simulink model "gabelstapler_Simulink"  (R2025a)
settings: Solver=VariableStepAuto  StartTime=0.0  StopTime=100  RelTol=1e-3
undefined symbols (not defined in the file): d_gtr, k_e, k_Motor, L_Motor, m_fz, m_gabel, R_Motor, r_R, theta_red
settings Model: Creator=Manuel  LastModifiedBy=baier

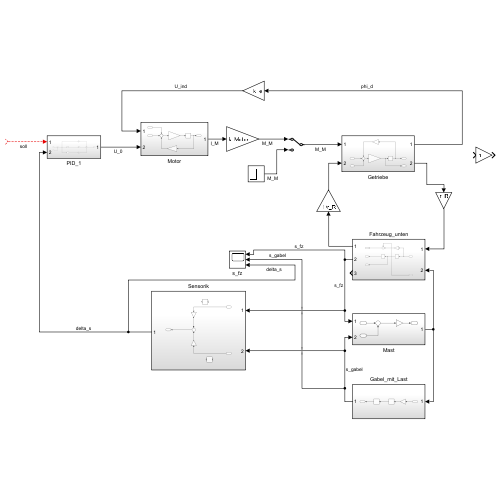
[thumbnail: Simulink's stored preview of the top-level diagram]
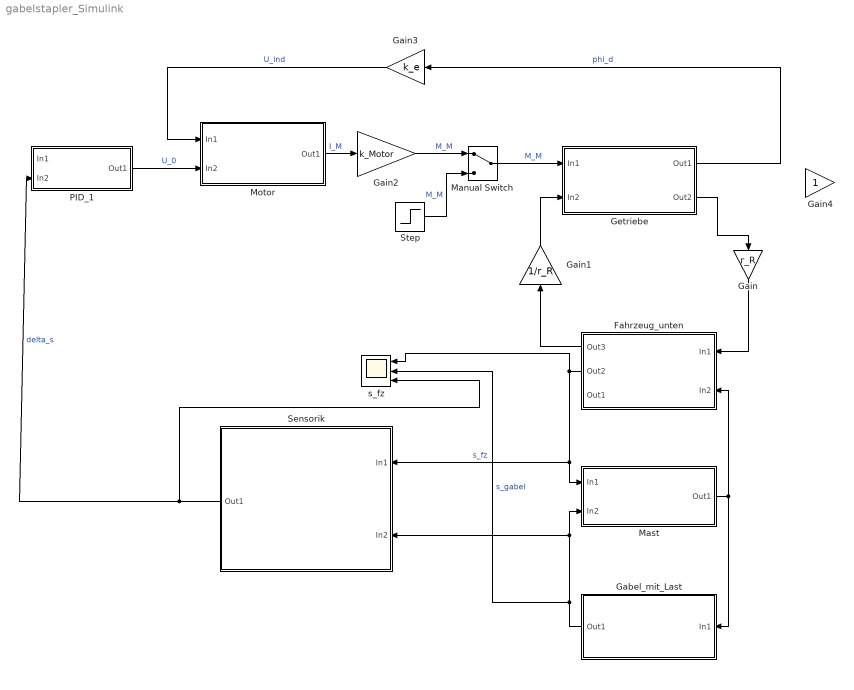
== system gabelstapler_Simulink ==
  Fahrzeug_unten : Subsystem
  Gabel_mit_Last : Subsystem
  Gain : Gain  Gain=r_R
  Gain1 : Gain  Gain=1/r_R
  Gain2 : Gain  Gain=k_Motor
  Gain3 : Gain  Gain=k_e
  Gain4 : Gain
  Getriebe : Subsystem
  Manual Switch : ManualSwitch
  Mast : Subsystem
  Motor : Subsystem
  PID_1 : Subsystem
  Sensorik : Subsystem
  Step : Step  SampleTime=0
  s_fz : Scope  NumInputPorts=3
      settings: ActiveDisplayYMinimum=-1.1492260881517071E+301  ActiveDisplayYMaximum=1.2769178757241187E+300
  wires:
  Gain3/1 -> Motor/1(In1)  "U_ind"
  PID_1/1(Out1) -> Motor/2(In2)  "U_0"
  Motor/1(Out1) -> Gain2/1  "I_M"
  Manual Switch/1 -> Getriebe/1(In1)  "M_M"
  Getriebe/1(Out1) -> Gain3/1  "phi_d"
  Getriebe/2(Out2) -> Gain/1
  Gain/1 -> Fahrzeug_unten/1(In1)
  Fahrzeug_unten/1(Out3) -> Gain1/1
  Gain1/1 -> Getriebe/2(In2)
  Fahrzeug_unten/2(Out2) -> Sensorik/1(In1), Mast/1(In1), s_fz/1  "s_fz"
  Gabel_mit_Last/1(Out1) -> s_fz/2, Mast/2(In2), Sensorik/2(In2)  "s_gabel"
  Mast/1(Out1) -> Gabel_mit_Last/1(In1), Fahrzeug_unten/2(In2)
  Sensorik/1(Out1) -> s_fz/3, PID_1/2(In2)  "delta_s"
  ? -> PID_1/1(In1)  "soll"
  Step/1 -> Manual Switch/2  "M_M"
  Gain2/1 -> Manual Switch/1  "M_M"

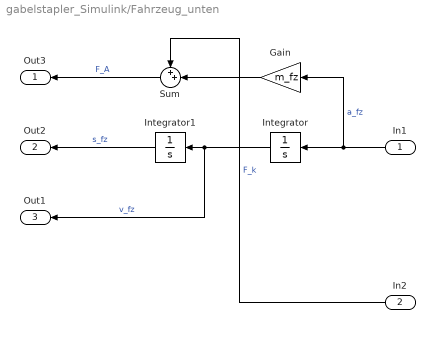
== system gabelstapler_Simulink/Fahrzeug_unten ==
  In1 : Inport
  In2 : Inport  Port=2
  Gain : Gain  Gain=m_fz
  Integrator : Integrator
  Integrator1 : Integrator
  Sum : Sum  Inputs=++|
  Out3 : Outport
  Out2 : Outport  Port=2
  Out1 : Outport  Port=3
  wires:
  Integrator/1 -> Out1/1, Integrator1/1  "v_fz"
  Integrator1/1 -> Out2/1  "s_fz"
  In1/1 -> Integrator/1, Gain/1  "a_fz"
  Sum/1 -> Out3/1  "F_A"
  In2/1 -> Sum/1  "F_k"
  Gain/1 -> Sum/2

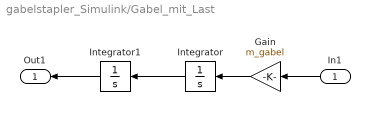
== system gabelstapler_Simulink/Gabel_mit_Last ==
  In1 : Inport
  Gain : Gain  Gain=m_gabel
  Integrator : Integrator
  Integrator1 : Integrator
  Out1 : Outport
  wires:
  Integrator/1 -> Integrator1/1
  In1/1 -> Gain/1
  Integrator1/1 -> Out1/1
  Gain/1 -> Integrator/1

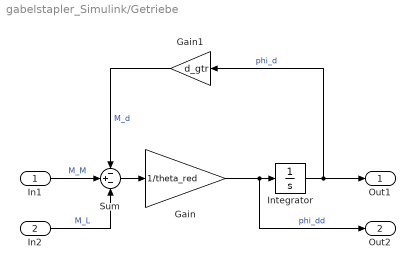
== system gabelstapler_Simulink/Getriebe ==
  In1 : Inport
  In2 : Inport  Port=2
  Gain : Gain  Gain=1/theta_red
  Gain1 : Gain  Gain=d_gtr
  Integrator : Integrator
  Sum : Sum  Inputs=-+-
  Out1 : Outport
  Out2 : Outport  Port=2
  wires:
  Sum/1 -> Gain/1
  Gain/1 -> Integrator/1, Out2/1  "phi_dd"
  Integrator/1 -> Out1/1, Gain1/1  "phi_d"
  Gain1/1 -> Sum/1  "M_d"
  In1/1 -> Sum/2  "M_M"
  In2/1 -> Sum/3  "M_L"

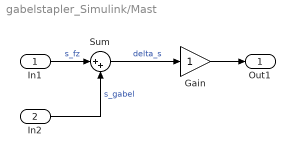
== system gabelstapler_Simulink/Mast ==
  In1 : Inport
  In2 : Inport  Port=2
  Gain : Gain
  Sum : Sum  Inputs=|++
  Out1 : Outport
  wires:
  Sum/1 -> Gain/1  "delta_s"
  In1/1 -> Sum/1  "s_fz"
  Gain/1 -> Out1/1
  In2/1 -> Sum/2  "s_gabel"

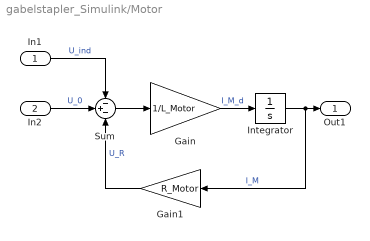
== system gabelstapler_Simulink/Motor ==
  In1 : Inport
  In2 : Inport  Port=2
  Gain : Gain  Gain=1/L_Motor
  Gain1 : Gain  Gain=R_Motor
  Integrator : Integrator
  Sum : Sum  Inputs=-+-
  Out1 : Outport
  wires:
  Gain1/1 -> Sum/3  "U_R"
  Sum/1 -> Gain/1
  In2/1 -> Sum/2  "U_0"
  In1/1 -> Sum/1  "U_ind"
  Integrator/1 -> Gain1/1, Out1/1  "I_M"
  Gain/1 -> Integrator/1  "I_M_d"

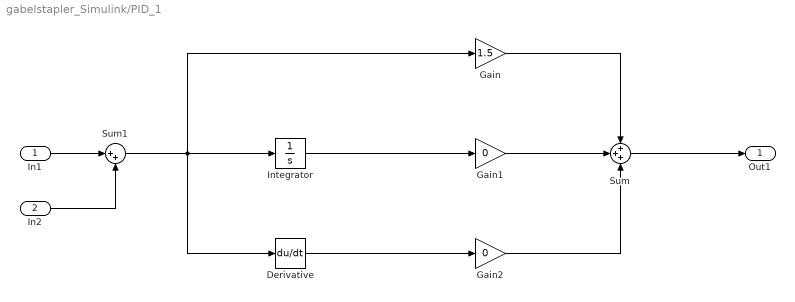
== system gabelstapler_Simulink/PID_1 ==
  In1 : Inport
  In2 : Inport  Port=2
  Derivative : Derivative
  Gain : Gain  Gain=1.5
  Gain1 : Gain  Gain=0
  Gain2 : Gain  Gain=0
  Integrator : Integrator
  Sum : Sum  Inputs=+++
  Sum1 : Sum  Inputs=|++
  Out1 : Outport
  wires:
  Integrator/1 -> Gain1/1
  Derivative/1 -> Gain2/1
  Gain1/1 -> Sum/2
  Gain/1 -> Sum/1
  Gain2/1 -> Sum/3
  Sum/1 -> Out1/1
  In1/1 -> Sum1/1
  Sum1/1 -> Integrator/1, Derivative/1, Gain/1
  In2/1 -> Sum1/2

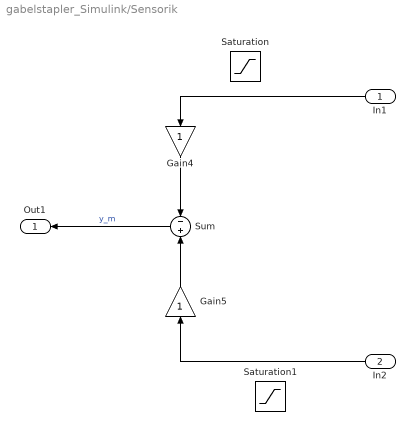
== system gabelstapler_Simulink/Sensorik ==
  In1 : Inport
  In2 : Inport  Port=2
  Gain4 : Gain
  Gain5 : Gain
  Saturation : Saturate
  Saturation1 : Saturate
  Sum : Sum  Inputs=-|+
  Out1 : Outport
  wires:
  In1/1 -> Gain4/1
  In2/1 -> Gain5/1
  Sum/1 -> Out1/1  "y_m"
  Gain5/1 -> Sum/2
  Gain4/1 -> Sum/1
